simulink model "Proyecto_labII_V1"  (R2025a)
settings: Solver=VariableStepAuto  StartTime=0.0  StopTime=10  RelTol=1e-3
settings Model: Creator=juand  LastModifiedBy=juand

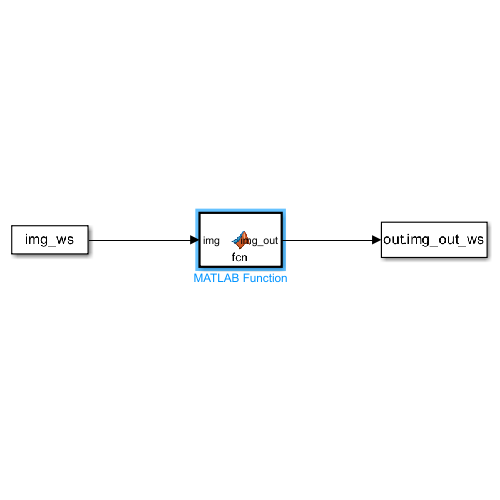
[thumbnail: Simulink's stored preview of the top-level diagram]
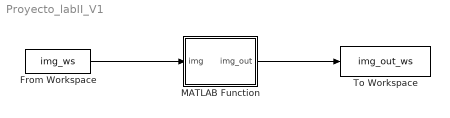
== system Proyecto_labII_V1 ==
  From Workspace : FromWorkspace  VariableName=img_ws  SampleTime=-1
  MATLAB Function : MATLAB Function  TreatAsAtomicUnit=on
  To Workspace : ToWorkspace  VariableName=img_out_ws  SaveFormat=Timeseries  SampleTime=-1
  wires:
  From Workspace/1 -> MATLAB Function/1(img)
  MATLAB Function/1(img_out) -> To Workspace/1

== matlab function Proyecto_labII_V1/MATLAB Function ==
  data: img input; img_out output
function img_out = fcn(img)
%#codegen
% Procesamiento básico de imagen RGB en Simulink

% Asegurar tipo double para procesamiento
img_d = double(img);

% Verificar que sea imagen RGB
if size(img_d,3) ~= 3
    error('La imagen no es RGB');
end

% Conversión a escala de grises (luminancia)
img_gray = 0.2989 * img_d(:,:,1) + ...
           0.5870 * img_d(:,:,2) + ...
           0.1140 * img_d(:,:,3);

% Volver a uint8 para visualización
img_out = uint8(img_gray);

end
